simulink model "AASHTO_Soil_Model"  (R2020a)
settings: Solver=VariableStepAuto  StartTime=0.0  StopTime=10.0  RelTol=1e-3
libraries: simulink x3
settings Model: Creator=SMONE  LastModifiedBy=SMONE

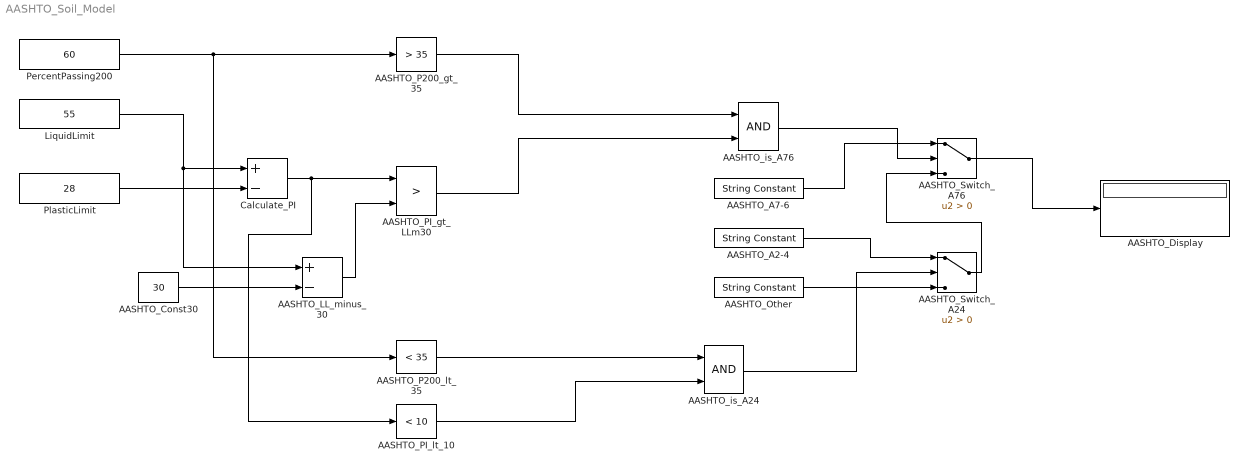
== system AASHTO_Soil_Model ==
  AASHTO_A2-4 : StringConstant  String='A-2-4'
  AASHTO_A7-6 : StringConstant  String='A-7-6'
  AASHTO_Const30 : Constant  Value=30
  AASHTO_Display : Display
  AASHTO_LL_minus_30 : Sum  Inputs=+-
  AASHTO_Other : StringConstant  String='AASHTO (Other)'
  AASHTO_P200_gt_35 : simulink/Logic and Bit Operations/Compare To Constant  relop=>  const=35  OutDataTypeStr=boolean
  AASHTO_P200_lt_35 : simulink/Logic and Bit Operations/Compare To Constant  relop=<  const=35  OutDataTypeStr=boolean
  AASHTO_PI_gt_LLm30 : RelationalOperator  Operator=>  OutDataTypeStr=boolean  RndMeth=Simplest
  AASHTO_PI_lt_10 : simulink/Logic and Bit Operations/Compare To Constant  relop=<  const=10  OutDataTypeStr=boolean
  AASHTO_Switch_A24 : Switch  Criteria=u2 > Threshold
  AASHTO_Switch_A76 : Switch  Criteria=u2 > Threshold
  AASHTO_is_A24 : Logic  AllPortsSameDT=off  OutDataTypeStr=boolean
  AASHTO_is_A76 : Logic  AllPortsSameDT=off  OutDataTypeStr=boolean
  Calculate_PI : Sum  Inputs=+-
  LiquidLimit : Constant  Value=55
  PercentPassing200 : Constant  Value=60
  PlasticLimit : Constant  Value=28
  wires:
  LiquidLimit/1 -> AASHTO_LL_minus_30/1, Calculate_PI/1
  PlasticLimit/1 -> Calculate_PI/2
  PercentPassing200/1 -> AASHTO_P200_gt_35/1, AASHTO_P200_lt_35/1
  AASHTO_Const30/1 -> AASHTO_LL_minus_30/2
  Calculate_PI/1 -> AASHTO_PI_gt_LLm30/1, AASHTO_PI_lt_10/1
  AASHTO_LL_minus_30/1 -> AASHTO_PI_gt_LLm30/2
  AASHTO_P200_gt_35/1 -> AASHTO_is_A76/1
  AASHTO_PI_gt_LLm30/1 -> AASHTO_is_A76/2
  AASHTO_P200_lt_35/1 -> AASHTO_is_A24/1
  AASHTO_PI_lt_10/1 -> AASHTO_is_A24/2
  AASHTO_Other/1 -> AASHTO_Switch_A24/3
  AASHTO_A2-4/1 -> AASHTO_Switch_A24/1
  AASHTO_is_A24/1 -> AASHTO_Switch_A24/2
  AASHTO_Switch_A24/1 -> AASHTO_Switch_A76/3
  AASHTO_A7-6/1 -> AASHTO_Switch_A76/1
  AASHTO_is_A76/1 -> AASHTO_Switch_A76/2
  AASHTO_Switch_A76/1 -> AASHTO_Display/1
